simulink model "HarmonicNLS_APF_Model"  (R2024a)
settings: Solver=VariableStepAuto  StartTime=0.0  StopTime=0.05  RelTol=1e-3
libraries: fl_lib x11, nesl_utility x6, ee_lib x2, slpidlib x1, spspowerguiLib x1
settings Model: Creator=divya  LastModifiedBy=h2kjp

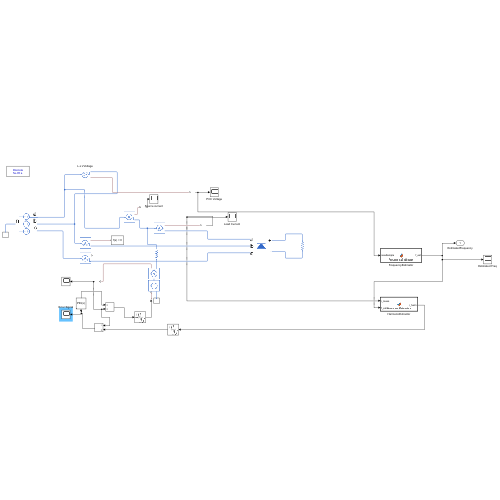
[thumbnail: Simulink's stored preview of the top-level diagram]
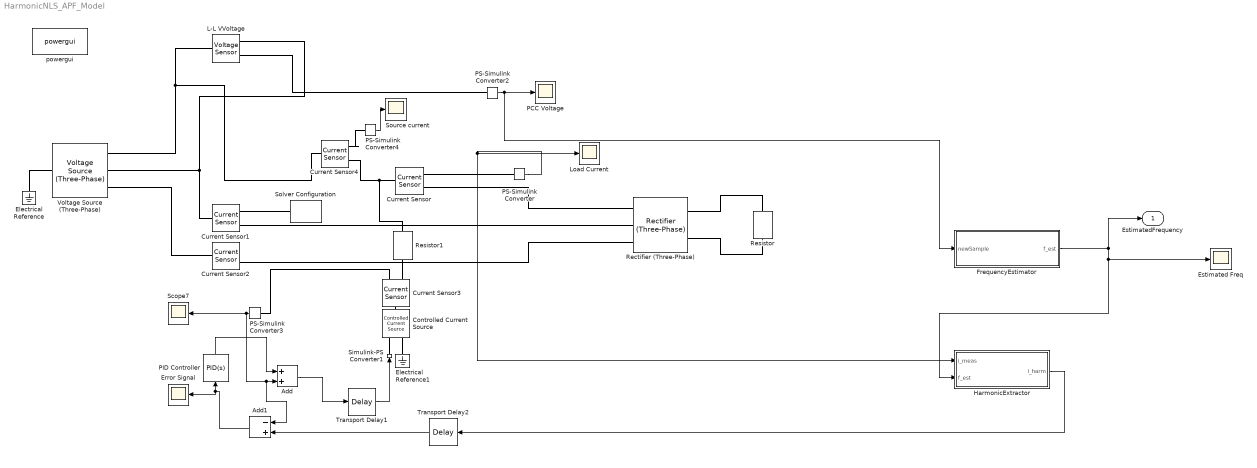
== system HarmonicNLS_APF_Model ==
  Add : Sum
  Add1 : Sum  Inputs=-+
  Controlled Current Source : fl_lib/Electrical/Electrical Sources/Controlled Current Source
  Current Sensor{,1..4} (5 alike) : fl_lib/Electrical/Electrical Sensors/Current Sensor
  Electrical Reference : fl_lib/Electrical/Electrical Elements/Electrical Reference
  Electrical Reference1 : fl_lib/Electrical/Electrical Elements/Electrical Reference
  Error Signal : Scope
  Estimated Freq : Scope
  FrequencyEstimator : MATLAB Function  TreatAsAtomicUnit=on  SystemSampleTime=0.000625
  HarmonicExtractor : MATLAB Function  TreatAsAtomicUnit=on  SystemSampleTime=0.0003125
  L-L VVoltage : fl_lib/Electrical/Electrical Sensors/Voltage Sensor
  Load Current : Scope
  PCC Voltage : Scope
  PID Controller : slpidlib/PID Controller  Controller=PID  Form=Parallel  TimeDomain=Continuous-time  UseExternalTs=off  SampleTime=-1  IntegratorMethod=Forward Euler  FilterMethod=Forward Euler  ControllerParametersSource=internal  P=.86  I=1e-1  UseKiTs=off  D=0  UseExternalDerivativeSource=off  N=100  UseFilter=on  TunerSelectOption=Transfer Function Based (PID Tuner App)  InitialConditionSource=internal  InitialConditionForIntegrator=0  InitialConditionForFilter=0  DifferentiatorICPrevScaledInput=0  ExternalReset=none  TrackingMode=off  Kt=1  LimitOutput=off  SatLimitsSource=internal  UpperSaturationLimit=inf  LowerSaturationLimit=-inf  LinearizeAsGain=on  AntiWindupMode=none  Kb=1  LimitIntegrator=off  UpperIntegratorSaturationLimit=inf  LowerIntegratorSaturationLimit=-inf  POutMin=[]  POutMax=[]  IOutMin=[]  IOutMax=[]  DOutMin=[]  DOutMax=[]  NOutMin=[]  NOutMax=[]  SumOutMin=[]  SumOutMax=[]  SaturationOutMin=[]  SaturationOutMax=[]  PParamMin=[]  PParamMax=[]  IParamMin=[]  IParamMax=[]  DParamMin=[]  DParamMax=[]  NParamMin=[]  NParamMax=[]  KbParamMin=[]  KbParamMax=[]  KtParamMin=[]  KtParamMax=[]  KbOutMin=[]  KbOutMax=[]  KtOutMin=[]  KtOutMax=[]  IntegratorOutMin=[]  IntegratorOutMax=[]  FilterOutMin=[]  FilterOutMax=[]  SumI1OutMin=[]  SumI1OutMax=[]  SumI2OutMin=[]  SumI2OutMax=[]  SumI3OutMin=[]  SumI3OutMax=[]  SumI4OutMin=[]  SumI4OutMax=[]  SumDOutMin=[]  SumDOutMax=[]  DifferentiatorOutMin=[]  DifferentiatorOutMax=[]  FilterDiffOutCoefMin=[]  FilterDiffOutCoefMax=[]  ReciprocalOutMin=[]  ReciprocalOutMax=[]  SumDenOutMin=[]  SumDenOutMax=[]  SumNumOutMin=[]  SumNumOutMax=[]  DivideOutMin=[]  DivideOutMax=[]  UdiffTsProdOutMin=[]  UdiffTsProdOutMax=[]  NTsProdOutMin=[]  NTsProdOutMax=[]  UintegralTsProdOutMin=[]  UintegralTsProdOutMax=[]  UngainTsProdOutMin=[]  UngainTsProdOutMax=[]  ClampingZeroOutDataTypeStr=Inherit: Inherit via back propagation  ClampingZeroOutMin=[]  ClampingZeroOutMax=[]  FilterDenConstantOutDataTypeStr=Inherit: Inherit via back propagation  FilterDenConstantOutMin=[]  FilterDenConstantOutMax=[]  PCopyOutDataTypeStr=Inherit: Inherit via back propagation  PCopyOutMin=[]  PCopyOutMax=[]  NCopyOutDataTypeStr=Inherit: Inherit via back propagation  NCopyOutMin=[]  NCopyOutMax=[]  IntegratorContinuousStateAttributes=''  IntegratorStateMustResolveToSignalObject=off  IntegratorRTWStateStorageClass=Auto  FilterContinuousStateAttributes=''  FilterStateMustResolveToSignalObject=off  FilterRTWStateStorageClass=Auto  ParallelPVariant=InternalParameters  IdealPVariant=Disabled  IVariant=InternalParameters  DVariant=InternalParameters  IntegratorVariant=Continuous  SatVariant=Disabled  AWVariant=Passthrough  PCopyVariant=Disabled  TRVariant=Disabled  FdbkBlocksVariant=Forward  IdealPFdbkVariant=Disabled  SatFdbkVariant=Disabled  DerivativeFilterVariant=ContFilter  NVariant=InternalParameters  NCopyVariant=Disabled  FilterICVariant=InternalICsFilter  IntegratorICVariant=InternalICs  ExternalResetVariant=Disabled  TRSumVariant=Passthrough  SumFdbkVariant=Disabled  SumVariant=Sum_PID  TsampFilterVariant=InternalTs  TsampNgainVariant=Passthrough  TsampIntegralVariant=Disabled_SignalSpec  ExternalSaturationOutDataTypeStr=Inherit: Same as second input  DerivativeSourceVariant=ErrorSignal
  PS-Simulink Converter{,2..4} (4 alike) : nesl_utility/PS-Simulink Converter  PhysicalDomain=network_engine_domain  SubClassName=ps_output  LeftPortType=input  RightPortType=output  PseudoPeriodic=off  Frequencies=[]  VectorFormat=inherit  Unit=inherit  AffineConversion=off
  Rectifier (Three-Phase) : ee_lib/Semiconductors & Converters/Converters/Rectifier (Three-Phase)  port_option=ee.enum.threePhasePort.expanded  Vf=0.8 V  Ron=0.001 Ohm  Goff=1e-5 1/Ohm  model_dynamics=ee.enum.converters.diode.nodynamics  C=50 nF  iRM=-235 A  iF=300 A  idot=-50 A/us  trr_param=ee.enum.converters.diodetrr.trr_factor  trr_factor=3  trr=15 us  Qrr=1500 s*uA
      settings: InternalSimscapePortConfiguration="{\"Bottom\":[],\"Left\":[{\"id\":\"a\",\"label\":\"a\",\"type\":\"foundation.electrical.electrical\"},{\"id\":\"b\",\"label\":\"b\",\"type\":\"foundation.electrical.electrical\"},{\"id\":\"c\",\"label\":\"c\",\"type\":\"foundation.electrical.electrical\"}],\"Right\":[{\"id\":\"p\",\"label\":\"+\",\"type\":\"foundation.electrical.electrical\"},{\"id\":\"n\",\"label\":\"-\",\"type\":\"foundation.electrical.electrical\"}],\"Top\":[]}"
  Resistor : fl_lib/Electrical/Electrical Elements/Resistor  R=20 Ohm  i_specify=off  i_priority=None  i=0 A  i_nominal_specify=off  i_nominal_value=1  i_nominal_unit=A  v_specify=off  v_priority=None  v=0 V  v_nominal_specify=off  v_nominal_value=1  v_nominal_unit=V
  Resistor1 : fl_lib/Electrical/Electrical Elements/Resistor  R=1e-3 Ohm  i_specify=off  i_priority=None  i=0 A  i_nominal_specify=off  i_nominal_value=1  i_nominal_unit=A  v_specify=off  v_priority=None  v=0 V  v_nominal_specify=off  v_nominal_value=1  v_nominal_unit=V
  Scope7 : Scope
  Simulink-PS Converter1 : nesl_utility/Simulink-PS Converter  PhysicalDomain=network_engine_domain  SubClassName=ps_input  LeftPortType=input  RightPortType=output  PseudoPeriodic=off  Frequencies=[]  NoiseDistribution=none  NoiseParameters=[]  Unit=1  AffineConversion=off  FilteringAndDerivatives=provide  SimscapeFilterOrder=1  InputFilterTimeConstant=0.001  UdotUserProvided=0
  Solver Configuration : nesl_utility/Solver Configuration  PhysicalDomain=network_engine_domain  SubClassName=solver  LeftPortType=input  RightPortType=generic  Tones=[]  Harmonics=[]  SimulateNoise=off  Profile=off  UseLocalSampling=off  EnableSwitchedLinearOptims=on  FrequencyDomain=off  UseCCode=off  RelTol=0.001  AbsTol=0.001  MinStep=1e-09  ToWorkspace=off  RevertToSquareIcSolve=off  NumHomotopyIterations=100  PhasorMode=off  PhasorModeNumHarmonics=1  ConsistencySolver=NEWTON_XTOL_AFTER_FTOL  IndexReductionMethod=DerivativeReplacement  DoDC=off  ResidualTolerance=1e-09  ConsistencyTolSource=GLOBAL  ConsistencyAbsTol=0.001  ConsistencyRelTol=0.001  ConsistencyTolFactor=0.001  UseLocalSolver=off  LocalSolverChoice=NE_BACKWARD_EULER_ADVANCER  ResolveIndetEquations=on  FunctionEvalNumThread=1  LocalSolverSampleTime=0.001  DoFixedCost=off  MaxNonlinIter=3  MaxModeIter=2  ComputeImpulses=off  ImpulseIterations=2  LinearAlgebra=auto  LinearAlgebraNumThread=0  EquationFormulation=NE_TIME_EF  DelaysMemoryBudget=1024  AutomaticFiltering=on  FilteringTimeConstant=0.001  PartitionStorageMethod=AS_NEEDED  PartitionMemoryBudget=1024  PartitionMethod=ROBUST  MultibodyUseLocalSolver=off  MultibodyLocalSolverChoice=ODE1  MultibodyLocalSolverSampleTime=0.001
  Source current : Scope
  Transport Delay1 : TransportDelay  DelayTime=1e-6
  Transport Delay2 : TransportDelay  DelayTime=1e-6
  Voltage Source (Three-Phase) : ee_lib/Sources/Voltage Source (Three-Phase)  vline_rms=sqrt(3) * 100 / sqrt(2) V  shift=0 deg  freq=50.8 Hz  impedance_option=0  SShortCircuit=1e6 A*V  XR=15  R=0.01 Ohm  L=3.97e-4 H  harmonic_option=0  harmonic_orders=[5, 7, 11, 13]  harmonic_ratios=[.1, .1, .1, .1]  G_parasitic=0 1/Ohm  I_specify=off  I_priority=None  I=[0, 0, 0] A  I_nominal_specify=off  I_nominal_value=1  I_nominal_unit=A
      settings: InternalSimscapePortConfiguration="{\"Bottom\":[],\"Left\":[{\"id\":\"n\",\"label\":\"n\",\"type\":\"foundation.electrical.electrical\"}],\"Right\":[{\"id\":\"a\",\"label\":\"a\",\"type\":\"foundation.electrical.electrical\"},{\"id\":\"b\",\"label\":\"b\",\"type\":\"foundation.electrical.electrical\"},{\"id\":\"c\",\"label\":\"c\",\"type\":\"foundation.electrical.electrical\"}],\"Top\":[]}"
  powergui : spspowerguiLib/powergui  Priority=1  SimulationMode=Discrete  SampleTime=50e-6  frequency=60  Iterations=50  frequencyindice=60  Pbase=100e6  ErrMax=1e-4  UnitsV=kV  UnitsW=MW  buscounter=0  FunctionMessages=off  echomessages=off  EnableUseOfTLC=off  CurrentSourceSwitches=off  DisableSnubberDevices=off  DisableRonSwitches=off  DisableVfSwitches=off  DisplayEquations=off  AutomaticDiscreteSolvers=off  SolverType=Tustin/Backward Euler (TBE)  Interpol=off  ExternalGateDelay=off  methode=off  Ts=100  x0status=blocks  SPID=on  SwTol=0  HookPort=off  NonlinearTolerance=1e-4  nMaxIteration=100  ContinueOnMaxIteration=off  RestoreLinks=warning  ResistiveCurrentMeasurement=off  Frange=[0:2:500]  Ylog=off  Xlog=on  ShowGrid=off  save=off  variable=ZData  structure=0  ZoomFFT=off  StartTime=0.0  cycles=1  DisplayStyle=1  fundamental=60  FreqAxis=off  MaxFrequency=1000  frequencyindicesteady=1  RmsSteady=1  display=off
  EstimatedFrequency : Outport
  wires:
  PS-Simulink Converter2/1 -> FrequencyEstimator/1(newSample), PCC Voltage/1
  PS-Simulink Converter/1 -> HarmonicExtractor/1(i_meas), Load Current/1
  HarmonicExtractor/1(i_harm) -> Transport Delay2/1
  FrequencyEstimator/1(f_est) -> HarmonicExtractor/2(f_est), Estimated Freq/1, EstimatedFrequency/1
  PS-Simulink Converter3/1 -> Add1/1, Add/2, Scope7/1
  Transport Delay1/1 -> Simulink-PS Converter1/1
  Transport Delay2/1 -> Add1/2
  PS-Simulink Converter4/1 -> Source current/1
  Add1/1 -> Error Signal/1, PID Controller/1
  PID Controller/1 -> Add/1
  Add/1 -> Transport Delay1/1
  connections:
  Voltage Source (Three-Phase)/LConn1 -- Electrical Reference/LConn1
  Rectifier (Three-Phase)/RConn1 -- Resistor/LConn1
  Rectifier (Three-Phase)/RConn2 -- Resistor/RConn1
  Voltage Source (Three-Phase)/RConn1 -- L-L VVoltage/LConn1 -- Current Sensor4/LConn1
  Voltage Source (Three-Phase)/RConn2 -- L-L VVoltage/RConn2 -- Current Sensor1/LConn1
  Current Sensor1/RConn2 -- Rectifier (Three-Phase)/LConn2
  Voltage Source (Three-Phase)/RConn3 -- Current Sensor2/LConn1
  Current Sensor2/RConn2 -- Rectifier (Three-Phase)/LConn3
  Current Sensor/RConn1 -- PS-Simulink Converter/LConn1
  L-L VVoltage/RConn1 -- PS-Simulink Converter2/LConn1
  Current Sensor/RConn2 -- Rectifier (Three-Phase)/LConn1
  Current Sensor3/RConn1 -- PS-Simulink Converter3/LConn1
  Solver Configuration/RConn1 -- Current Sensor1/RConn1
  Resistor1/LConn1 -- Current Sensor3/RConn2
  Simulink-PS Converter1/RConn1 -- Controlled Current Source/RConn1
  Electrical Reference1/LConn1 -- Controlled Current Source/RConn2
  Controlled Current Source/LConn1 -- Current Sensor3/LConn1
  Resistor1/RConn1 -- Current Sensor4/RConn2 -- Current Sensor/LConn1
  Current Sensor4/RConn1 -- PS-Simulink Converter4/LConn1

== matlab function HarmonicNLS_APF_Model/FrequencyEstimator ==
  data: newSample input; f_est output
function f_est = FrequencyEstimator(newSample)
newSample
%#codegen
% FrequencyEstimator estimates the fundamental frequency using a 
% nonlinear least-squares (NLS) method with harmonic terms.
%
% The measured signal is modeled as a Fourier series:
%    v(t) ≈ sum_{h in allowed_harmonics} [ a_h*sin(2*pi*f*h*t) + b_h*cos(2*pi*f*h*t) ]
%
% This function accumulates a window of samples and then searches over a range
% of candidate frequencies to find the frequency f that minimizes the sum of squared
% errors between the measured window and the model.
%
% Inputs:
%   newSample - The new measured sample (scalar)
%
% Output:
%   f_est     - Estimated fundamental frequency (Hz)
%
% Note: Adjust Ts and N_window as necessary.

% Persistent variables to store the sample buffer, counter, and parameters
persistent buffer sampleCount Ts N_window f_prev allowed_harmonics
if isempty(sampleCount)
    Ts = 1/1600;          % Sampling period (for 1.6 kHz sampling rate)
    N_window = 16;        % Window length in samples (approx. one cycle at 50 Hz)
    buffer = zeros(N_window, 1);  % Preallocate buffer
    sampleCount = 0;
    f_prev = 50;          % Initial frequency guess (Hz)
    allowed_harmonics = [1, 5, 7, 11, 13]; % Selected harmonics to include in the model
end

% Accumulate samples until the buffer is full; then use a sliding window.
if sampleCount < N_window
    sampleCount = sampleCount + 1;
    buffer(sampleCount) = newSample;
    f_est = f_prev;   % Until the window is full, output the previous estimate.
    return;
else
    % Slide the window by one sample and append the new sample
    buffer(1:end-1) = buffer(2:end);
    buffer(end) = newSample;
end

% Create a time vector for the current window (relative time starting at 0)
t_window = ((0:N_window-1)' * Ts);

% Define candidate frequency range (e.g., around nominal 50 Hz)
f_candidates = 30:0.01:70;  % Hz

minError = inf;
f_best = f_prev; % Default value

% Iterate over candidate frequencies
for f = f_candidates
    % Build the regression matrix including the selected harmonics
    % For each harmonic h, add columns for sin(2*pi*f*h*t) and cos(2*pi*f*h*t)
    M = [];
    for hh = allowed_harmonics
        M = [M, sin(2*pi*f*hh*t_window), cos(2*pi*f*hh*t_window)]; %#ok<AGROW>
    end
    
    % Solve the linear least-squares problem for the coefficient vector
    coeff = (M'*M)\(M'*buffer);
    
    % Reconstruct the signal over the window using the estimated coefficients
    buffer_est = M * coeff;
    
    % Compute the sum of squared errors (SSE)
    err = sum((buffer - buffer_est).^2);
    
    % If error is lower, update the best frequency estimate
    if err < minError
        minError = err;
        f_best = f;
    end
end

% Update persistent frequency guess and output the best candidate
f_prev = f_best;
f_est = f_best
f_best

== matlab function HarmonicNLS_APF_Model/HarmonicExtractor ==
  data: i_meas input; i_harm output; f_est input
function i_harm = HarmonicEstimator(i_meas, f_est)
%#codegen
%
% HarmonicEstimator:
%   Implements the method from the research paper to estimate the 
%   fundamental component of i_meas using a Fourier series model that
%   includes multiple harmonic orders, and then extracts the harmonic 
%   component as:
%
%       i_harm = i_meas - i_fund.
%
% The model uses a sliding window of ~10 ms (N_window samples) and a persistent 
% buffer to store the last N_window samples.
%
% The regression matrix H is constructed using the estimated frequency f_est 
% and the allowed harmonic orders. Here we use:
%       allowed_harmonics = [1, 3, 5, 7, 9, 11, 13]
%
% For each harmonic h, two columns are added:
%   sin(2*pi*f_est*h*t) and cos(2*pi*f_est*h*t).
%
% The coefficient vector is then computed as:
%       x = (H' * H)^(-1) * H' * buffer,
%
% from which the fundamental component (h = 1) is reconstructed using the first
% two coefficients. Finally, the harmonic component is computed by subtracting the 
% fundamental component from the measured sample.
%
% Inputs:
%   i_meas : (scalar) New measured sample of current.
%   f_est  : (scalar) Estimated fundamental frequency (Hz).
%
% Output:
%   i_harm : (scalar) Harmonic component = i_meas - i_fund.

%% Persistent Variables
persistent buffer sampleCount Ts N_window allowed_harmonics
if isempty(sampleCount)
    Ts = 1/1600;% Sampling period for 1.6 kHz
    Ts=Ts/2;
    N_window = round(0.01 * 1/Ts);     % 10 ms window, approximately 16 samples
    buffer = zeros(N_window, 1);       % Initialize buffer
    sampleCount = 0;
    % Use allowed harmonics: fundamental and odd non-triplen harmonics.
    allowed_harmonics = [1, 3, 5, 7, 9, 11, 13, 15, 17];
end

%% Accumulate Samples in the Sliding Window
if sampleCount < N_window
    sampleCount = sampleCount + 1;
    buffer(sampleCount) = i_meas;
    i_harm = 0;  % Until the window is full, output 0 (or previous estimate)
    return;
else
    % Shift the buffer by one sample and add the new sample
    buffer(1:end-1) = buffer(2:end);
    buffer(end) = i_meas;
end

%% Build Time Vector for the Window
t_window = (0:N_window-1)' * Ts;

%% Construct Regression Matrix H Using All Allowed Harmonics
% Each harmonic h contributes two columns: sin(2*pi*f_est*h*t) and cos(2*pi*f_est*h*t)
H = [];
for h = allowed_harmonics
    H = [H, sin(2*pi*f_est*h*t_window), cos(2*pi*f_est*h*t_window)]; %#ok<AGROW>
end

%% Compute Coefficient Vector Using Normal Equations
% x = (H'*H)^(-1) * H' * buffer
M = H' * H;
rhs = H' * buffer;
x = M \ rhs;  % More numerically stable than using inv()

%% Reconstruct the Fundamental Component (h = 1)
% The first two columns of H correspond to h = 1.
t_last = t_window(end);            % Time corresponding to the last sample in the window
omegaFund = 2 * pi * f_est * 1;      % Angular frequency for the fundamental (h=1)
sinFund = sin(omegaFund * t_last);
cosFund = cos(omegaFund * t_last);
a1 = x(1);   % Coefficient corresponding to sin(2*pi*f_est*t)
b1 = x(2);   % Coefficient corresponding to cos(2*pi*f_est*t)
i_fund = a1 * sinFund + b1 * cosFund;

%% Compute the Harmonic Component
i_harm = i_meas - i_fund;
